simulink library "carnot"  (R2018b)
settings: Solver=VariableStepAuto  StartTime=0.0  StopTime=10.0  RelTol=1e-3
undefined symbols (not defined in the file or in its folder): A, A_earth, acol, Acol, ActPower1, ActPower2, ActPower3, Ad, Ad0, Ar, Au, Au0, Azimuth_Angle, B, Bd, Bd0, Br, Bu, Bu0, C, c1, c2, c3, c33, c4, c5, c6, CarnotCallbacks_Density, CarnotCallbacks_Enthalpy, CarnotCallbacks_Enthalpy2Temperature, CarnotCallbacks_Entropy, CarnotCallbacks_Evaporation_Enthalpy, CarnotCallbacks_GlobalMessageLevel, CarnotCallbacks_Grashof, CarnotCallbacks_Heat_Capacity, CarnotCallbacks_Kinematic_Viscosity, CarnotCallbacks_PMV_PPD, CarnotCallbacks_Prandtl, CarnotCallbacks_Saturation_Property, CarnotCallbacks_Saturation_Temperature, CarnotCallbacks_Saturation_Value_Water, CarnotCallbacks_Specific_Volume, CarnotCallbacks_Thermal_Conductivity, CarnotCallbacks_Vapour_Content, CarnotCallbacks_Vapour_Pressure, Cd, Cdl, Cr, Cu, Davies, Dd, DE_TRY2010_04_averageYear, delta_grd, density, DiameterLastPiece, dl, DPConstant, DPLinear, DPQuadratic, Dr ... (+59)
libraries: $bdroot x429, simulink x36, simulink_extras x12
(part 1 of 22)
settings Model: Creator=P41573  LastModifiedBy=drhf

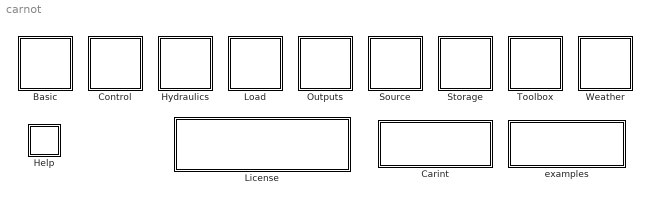
== system carnot ==
  Basic : Subsystem
      mask Display: plot(0,0,100,100,[10,10,40,40,10],[10,40,40,10,10],[50,70,90,50],[30,65,30,30],[20,10,10,20,30,40,40,30,20],[50,60,70,80,80,70,60,50,50])
  Carint : Subsystem
      settings: OpenFcn=carint
      mask Display: disp('double click to\nload Carnot Internal');
  Control : Subsystem
      mask Display: plot(0,0,100,100,[70,100,40,10,70,70,10,10],[50,80,80,50,50,20,20,50],[100,70],[50,20],[20,50,50,20,20],[40,40,30,30,40],[62,62,62,61,59,58,58,60],[42,41,39,38,38,40,42,43],[61,62,62,61,60,59,58,58,58,59],[32,31,30,28,27,28,28,30,31,32])
  Help : Subsystem
      settings: OpenFcn=helpcarnot
      mask Display: disp('?');
  Hydraulics : Subsystem
      mask Display: plot(0,0,100,100,[15,18,18,15,40,40,46,55,60,60,55,46,40,40,15,10,10,15],[60,53,46,40,40,20,24,24,20,80,85,85,80,60,60,53,46,40],[60,55,46,40],[20,15,15,20])
  License : Subsystem
      mask Display: disp('Carnot 7.3\nfor MATLAB R2018b\nCopyright Solar-Institute Juelich');
  Load : Subsystem
      mask Display: plot(0,0,100,100,[10,20,30,10,30,30,10,10],[30,50,30,30,30,10,10,30],[30,20,10,30,30,10,10],[80,100,80,80,60,60,80],[77,76,70,50],[70,76,80,80],[74,66],[90,90],[70,70],[80,89],[77,76,70,50],[20,26,30,30],[74,66],[40,40],[70,70],[30,39])
  Outputs : Subsystem
      mask Display: plot(0,0,100,100,[90,10,10],[10,10,90],[90,80,70,60,50,10],[65,63,50,26,20,20],[90,70,57,46,40,31,40,50,60,70,90],[78,78,72,60,36,20,20,33,60,70,70],[90,60,45,31,24,21,14,21,30,34,44,59,90],[87,87,85,75,58,35,20,20,37,58,77,83,83])
  Source : Subsystem
      mask Display: plot(0,0,100,100,[30,40,60,70,70,30,30],[50,44,44,50,10,10,50],[50,50],[44,57],[50,46,44,46,50,54,56,54,50],[93,85,70,54,48,54,70,85,93])
  Storage : Subsystem
      mask Display: plot(10,10,90,100,[40,40,45,55,60,60,55,45,40],[84,36,30,30,36,84,90,90,84],[40,35],[77,77],[64,60],[77,77],[40,35],[42,42],[64,60],[42,42])
  Toolbox : Subsystem
      mask Display: plot(0,0,100,100,[10,40,50,40,10,10],[90,90,80,70,70,90],[28,28,22,22],[70,10,10,70],[70,80,80,70,70],[50,50,10,10,50],[77,77],[10,50],[73,73],[10,50],[76,76,74,74],[50,90,90,50])
  Weather : Subsystem
      mask Display: plot(7,7,95,100,[10,7,10,20,30,23,25,40,54,56,50,60,70,73,70,60,20,10],[15,24,34,40,35,42,50,55,50,42,35,40,34,24,15,10,10,15],[70,60,60,70,80,90,90,80,70],[90,80,70,60,60,70,80,90,90],[75,75],[91,97],[75,75],[52,58],[58,52],[75,75],[98,91],[75,75],[63,58],[63,57],[92,86],[92,87],[63,58],[85,92],[92,86],[57,64])
  examples : Subsystem
      settings: OpenFcn=CarnotCallbacks_LoadExamples
      mask Display: disp('double click \nto load examples');

== system carnot/Basic ==
  Electric : Subsystem
      mask Display: plot(0,0,100,100,[40,20],[50,50],[40,40],[30,70],[50,50],[-0,100],[70,50],[50,50])
  Heat_Transfer : Subsystem
      mask Display: plot(0,0,100,100,[50,50],[-0,100],[30,40,49,49,40,30],[10,20,41,60,80,90],[40,30,30],[10,10,20],[70,60,52,51,60,70],[90,80,60,40,20,10],[70,70,60],[80,90,91])
  Hydraulics : Subsystem
      mask Display: plot(0,0,100,100,[15,18,18,15,40,40,46,55,60,60,55,46,40,40,15,10,10,15],[60,53,46,40,40,20,24,24,20,80,85,85,80,60,60,53,46,40],[60,55,46,40],[20,15,15,20])
  Material_Properties : Subsystem
      mask Display: plot(10,10,80,80,[30,25,20,25,30,30,40,40,25,10,10,20,20],[60,59,60,61,60,50,32,30,27,30,32,50,60],[50,54,54,50,60,68,70,60,50,45,40,40,44,50],[60,64,70,72,70,67,70,75,77,77,73,65,60,60],[70,65,60,65,70,70,67,64,60],[50,51,50,48,50,15,10,10,15],[60,60],[15,50])
  Pressure_Drop : Subsystem
      mask Display: plot(-20,10,60,100,[-20,-20,10,20,30,35,35,30,20,10,-20],[70,40,40,45,45,40,70,65,65,70,70],[55,37],[84,65],[56,37],[68,60],[56,37],[56,56],[55,37],[48,53],[54,37],[39,48],[50,37],[32,44],[44,37],[83,69],[44,37],[30,40])
  Thermal_Models : Subsystem
      mask Display: plot(-20,0,120,100,[10,70,70,10,10],[10,10,70,70,10],[70,90,90,30,10],[10,30,90,90,70],[90,70],[90,70],[50,30],[60,60],[40,40],[30,60])
  Weather_and_Sun : Subsystem
      mask Display: plot(7,7,95,100,[10,7,10,20,30,23,25,40,54,56,50,60,70,73,70,60,20,10],[15,24,34,40,35,42,50,55,50,42,35,40,34,24,15,10,10,15],[70,60,60,70,80,90,90,80,70],[90,80,70,60,60,70,80,90,90],[75,75],[91,97],[75,75],[52,58],[58,52],[75,75],[98,91],[75,75],[63,58],[63,57],[92,86],[92,87],[63,58],[85,92],[92,86],[57,64])

== system carnot/Carint ==

== system carnot/Control ==
  Controller_Bang_Bang : Subsystem  mask(bang bang controler){deltaTon=5, deltaToff=1, Tmax=95}
      mask prompts: deltaTon "deltaT-on [K]"; deltaToff "deltaT-off [K]"; Tmax "maximum temperature [degree centigrade]"
      mask help:
      | Hysteresis controller for thermal systems. Output is set to zero if Thot or Tcold is bigger than Tmax.
      | deltaT = Thot - Tcold
      mask Help: web(fullfile(path_carnot('help'),'Controller_Bang_Bang.html'),'-helpbrowser')
      mask Display: plot(-30,0,150,100,[70,100,40,10,70,70,10,10],[50,80,80,50,50,20,20,50],[100,70],[50,20],[20,50,50,20,20],[40,40,30,30,40],[62,62,62,61,59,58,58,60],[42,41,39,38,38,40,42,43],[61,62,62,61,60,59,58,58,58,59],[32,31,30,28,27,28,28,30,31,32])
  EnergyMeter : Subsystem  mask(energy meter){}
      mask help: Calculates the power and energy of a fluid flow between inlet and outlet of components.
      mask Help: web(fullfile(path_carnot('help'),'EnergyMeter.html'),'-helpbrowser')
  EnergyMeter_HC : Subsystem  mask(energy meter Heating/Cooling){}
      mask help:
      | Calculates the power and energy of a fluid flow between inlet and outlet of components.
      | Positive power is integrated to the heating energy, negative power is integrated to the cooling energy.
      mask Help: eval('htmlhelp (''chap_4_2e.htm#energy_meter'')');
  Massflow_Sensor : Subsystem  mask(temperature measurement sensor){tc=10, t0=0}
      mask prompts: tc "time constant of sensor [s]"; t0 "initial value [kg/s]"
      mask help: Measurement sensor for temperatures with first-oder hold. Temperature is in degree centigrade.
      mask init:
      | tc = 1/max(tc, 0.001);
      mask Help: web(fullfile(path_carnot('help'),'Massflow_Sensor.html'),'-helpbrowser')
  Max_Run_Time : Subsystem  mask(Maximum Running Time){tmaxrun=5}
      mask prompts: tmaxrun "Maximum operation time in s"
      mask help: Keeps the output to the input level until either the maximum running time is reached or the input is set to zero.
      mask Help: web(fullfile(path_carnot('help'),'Max_Run_Time.html'),'-helpbrowser')
      mask Display:
      | plot(-20,-30,120,100,[10,20,40,60,80,90,90,80,60,40,20,10,10],[40,20,10,10,20,40,60,80,90,90,80,60,40],[55,46],[95,95],[50,50],[90,95],[50,50,24],[88,50,66],[10,13],[50,50],[90,87],[50,50],[50,50],[10,15])
      | disp('\n\nMax On')
  Min_Run_Time : Subsystem  mask(Minimum Running Time){tminrun=2, mv=2}
      mask prompts: tminrun "Minimum operation time in s"; mv "Minimum output value"
      mask help: Once started, the output is kept to the maximum of the input value and the mimimum output for at least the minimum running time.
      mask Help: web(fullfile(path_carnot('help'),'Min_Run_Time.html'),'-helpbrowser')
      mask Display:
      | plot(-20,-30,120,100,[10,20,40,60,80,90,90,80,60,40,20,10,10],[40,20,10,10,20,40,60,80,90,90,80,60,40],[55,46],[95,95],[50,50],[90,95],[50,50,24],[88,50,66],[10,13],[50,50],[90,87],[50,50],[50,50],[10,15])
      | disp('\n\nMin On')
  Min_Stop_Time : Subsystem  mask(Minimum Stop Time){tminstop=15}
      mask prompts: tminstop "Minimum stop time in s"
      mask help: Once stopped, the output is held to zero for at least the minimum stop time.
      mask Help: web(fullfile(path_carnot('help'),'Min_Stop_Time.html'),'-helpbrowser')
      mask Display:
      | plot(-20,-30,120,100,[10,20,40,60,80,90,90,80,60,40,20,10,10],[40,20,10,10,20,40,60,80,90,90,80,60,40],[55,46],[95,95],[50,50],[90,95],[50,50,24],[88,50,66],[10,13],[50,50],[90,87],[50,50],[50,50],[10,15])
      | disp('\n\nMin Off')
  OnOff_switch : Constant  Value=0
      settings: OpenFcn=set_param(gcb,'value',num2str(1-str2num(get_param(gcb,'value'))))
      mask Help: web(fullfile(path_carnot('help'),'OnOff_Switch.html'),'-helpbrowser')
  PowerMeter : Subsystem  mask(power meter){}
      mask help:
      | Calculates the power of a fluid flow between inlet and outlet of components characterized by the THB.
      | Qdot = mdot * cp(Tmean) * (Tout - Tin)
      | Tmean = (Tin+Tout)/2
      mask Help: web(fullfile(path_carnot('help'),'PowerMeter.html'),'-helpbrowser')
  Shading_Control : Subsystem  mask(Shading Control){TroomShadeOn=23.8, TroomShadeOff=22.8, SolarShadeOn=300, SolarShadeOff=200, max_shade=1}
      mask prompts: TroomShadeOn "Room temperature to switch shading on in °C"; TroomShadeOff "Room temperature to switch shading off in °C"; SolarShadeOn "Solar radiation to switch shading on in W/m²"; SolarShadeOff "Solar radiation to switch shading off in W/m²"; max_shade "Maximum value for Sunshade"
      mask help:
      | Active the Sunshade of a window when:
      | + room temperature is above shading temperture
      | + outdoor ambient temperature is above 10°C
      | + solar radiation is above 300 W/m²
      | The solar gains of a window is:
      | SolarGain = LightTransmittance * WindowSurface
      |                     * SolarRadiation * (1 - Sunshade)
      mask TypeOptions TroomShadeOn: Hyst_Troom/OnSwitchValue
      mask TypeOptions TroomShadeOff: Hyst_Troom/OffSwitchValue
      mask TypeOptions SolarShadeOn: Hsyt_Solar/OnSwitchValue
      mask TypeOptions SolarShadeOff: Hsyt_Solar/OffSwitchValue
      mask TypeOptions max_shade: Saturation/UpperLimit
      mask Display:
      | plot(0,-5,100,95,...
      |     [70,60,60,70,80,90,90,80,70],[90,80,70,60,60,70,80,90,90],...
      |     [75,75],[91,95],[75,75],[52,58],[58,52],[75,75],...
      |     [98,91],[75,75],[63,58],[63,57],[92,86],[92,87],...
      |     [63,58],[85,92],[92,86],[57,64], ...
      |     [10,20,30,37,41,48,50,10],[51,53,53,51,45,31,20,51],...
      |     [33,30],[0,35])
  Solar_Radiation_Sensor : Subsystem  mask(measure solar radiation){rad=diffuse, rad_typ=normal to the beam radiation}
      mask prompts: rad "measured radiation"; rad_typ "orientation of the sensor"
      mask help:
      | Extracts the solar radiation in W/m² from the weather data vector.
      |
      | WARNING:
      | For old weather data vectors, their is only one type of tsolar radiation.
      mask init:
      | if (rad_typ == 1)
      |     if (rad == 1)
      |         vector = [3];
      |     elseif (rad == 2)
      |         vector = [4];
      |     else
      |         vector = [3 4];
      |     end
      | else
      |     if (rad == 1)
      |         vector = [16];
      |     elseif (rad == 2)
      |         vector = [17];
      |     else
      |         vector = [16 17];
      |     end
      | end
      mask Help: web(fullfile(path_carnot('help'),'Solar_Radiation_Sensor.html'),'-helpbrowser')
      mask TypeOptions rad: direct | diffuse | global
      mask TypeOptions rad_typ: normal to the beam radiation | fixed (horizontal or inclined)
  Start_Delay : Subsystem  mask(Start Delay){tstartdelay=5}
      mask prompts: tstartdelay "Start delay time in s"
      mask help: The output is delayed for the delay time, than it equal to the input.
      mask Help: web(fullfile(path_carnot('help'),'Start_Delay.html'),'-helpbrowser')
      mask Display:
      | plot(-20,-30,120,100,[10,20,40,60,80,90,90,80,60,40,20,10,10],[40,20,10,10,20,40,60,80,90,90,80,60,40],[55,46],[95,95],[50,50],[90,95],[50,50,24],[88,50,66],[10,13],[50,50],[90,87],[50,50],[50,50],[10,15])
      | disp('\n\nDelay On')
  T_Sensor : Subsystem  mask(temperature measurement sensor){tc=10, t0=20}
      mask prompts: tc "time constant of sensor [s]"; t0 "initial temperature [degree centigrade]"
      mask help: Measurement sensor for temperatures with first-oder hold. Temperature is in degree centigrade.
      mask init:
      | tc = 1/max(tc, 0.001);
      mask Help: web(fullfile(path_carnot('help'),'T_Sensor.html'),'-helpbrowser')
      mask Display: plot(0,0,100,100,[50,55,65,70,70,65,55,45,35,30,30,35,44,50,50],[50,50,60,70,80,90,100,100,90,80,70,60,50,50,-0],[60,40],[90,90],[50,50],[57,90])
  T_Sensor_Surface : Subsystem  mask(surface temperature sensor){pos=[0.1 0.4 0.5 0.9], tdel=1, t0=20}
      mask prompts: pos "relative position 0..1 (0 = bottom, 1 = top)"; tdel "delay-time in s"; t0 "initial temperature in degree centigrade"
      mask help:
      | Surface temperature sensor for a storage. The block breaks the algebraic loop when connecting the node temperature directly to the controller.
      | The relative position can be a vector for several sensors, for example [0.1 0.5 0.9]
      mask init:
      | tdel = max(tdel,0.01);
      | pos = max(0, min(pos, 1));
      mask Help: web(fullfile(path_carnot('help'),'T_Sensor_Surface.html'),'-helpbrowser')
      mask Display: plot(-10,0,110,100,[50,55,65,70,70,65,55,45,35,30,30,35,44,50,50],[50,50,60,70,80,90,100,100,90,80,70,60,50,50,-0],[60,40],[90,90],[50,50],[57,90])
  Thermostat_Proportional : Subsystem  mask(Thermostat){op=0.5, bl=0.2, p=4, ts=60}
      mask prompts: op "Operation point (valve position at set temperature)"; bl "Hysteresis or play in K"; p "Proportional range in K"; ts "First order hold for temperature sensor in s"
      mask help: Thermostat with proportional characteristic and play.
      mask TypeOptions op: operationPosition/Value
      mask TypeOptions bl: Play/Value | Backlash/BacklashWidth
      mask TypeOptions p: proportionalRange/Value
      mask TypeOptions ts: Sensor/ts
      mask Display: plot(-10,15,80,95,[10,20,30,40,40,30,20,10,10],[30,20,20,30,40,50,50,40,30],[40,60,60,50,40,30,10],[30,70,80,90,90,80,40],[50,30],[90,50],[60,40],[80,41],[40,20],[90,50],[19,11,14],[36,36,33],[23,26,29,29,25,28,23],[41,39,41,43,45,48,48],[32,31,32,35,35,38,38],[39,36,33,35,39,39,33])
  Window_Control : Subsystem  mask(Window Control){Topen=24, Tclose=23, TrAboveTa=2, TaTooCold=12, timeFIR=24, TaIni=12, starttime=8, stoptime=22}
      mask prompts: Topen "Open window if Troom is above [°C]"; Tclose "Close window if Troom is below [°C]"; TrAboveTa "Open window if Troom is above Tamb [K]"; TaTooCold "Close window if Tamb is below [°C]"; timeFIR "Average time for Tamb in h (only integer values)"; TaIni "Initial value for Tamb in °C"; starttime "Start time in the morning [h]"; stoptime "Stop time in the evening [h]"
      mask help:
      | Control for free driven passive cooling realized by tilted windows.
      | Window is opened if:
      | + Room temperature (Troom) is above a fixed value
      | + Outdoor ambient temperature (Tamb) is below Troom
      | + Average of Tamb is not too cold
      | + During the day (starttime <= time < stoptime)
      mask Help: web(fullfile(path_carnot('help'),'Window_Control.html'),'-helpbrowser')
      mask TypeOptions Topen: RelayTroom/OnSwitchValue
      mask TypeOptions Tclose: RelayTroom/OffSwitchValue
      mask TypeOptions TrAboveTa: Troom_GE_Tamb/const
      mask TypeOptions TaTooCold: Tamb_GT_Const/const
      mask TypeOptions TaIni: MovingAverage/InitialStates
      mask TypeOptions starttime: FromMorning/const
      mask TypeOptions stoptime: TillEvening/const
      mask Display:
      | plot(-5,10,90,80,[20 70 70 20 20],[20 20 70 70 20],...
      |     [20 70 80 30 20],[20 20 65 65 20])

== system carnot/Help ==
